simulink model "fymohukongzhifangzhen"  (R2012b)
settings: Solver=ode3  StartTime=0.0  StopTime=10.0  FixedStep=0.005  RelTol=1e-3
libraries: fuzblock x1
settings Model: Creator=Administrator  LastModifiedBy=Administrator

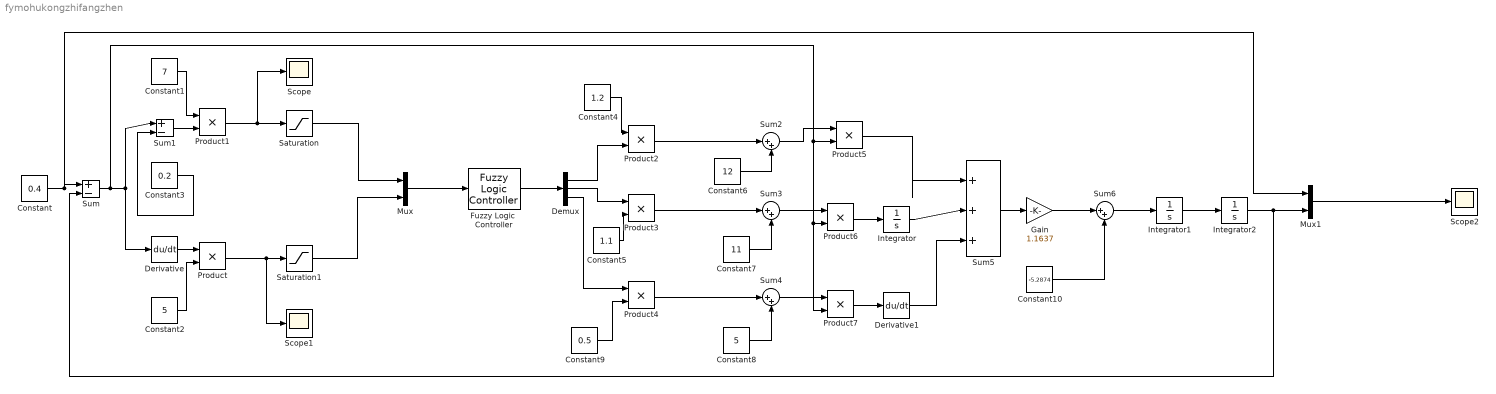
== system fymohukongzhifangzhen ==
  Constant : Constant  Value=0.4
  Constant1 : Constant  Value=7
  Constant10 : Constant  Value=-5.2874
  Constant2 : Constant  Value=5
  Constant3 : Constant  Value=0.2
  Constant4 : Constant  Value=1.2
  Constant5 : Constant  Value=1.1
  Constant6 : Constant  Value=12
  Constant7 : Constant  Value=11
  Constant8 : Constant  Value=5
  Constant9 : Constant  Value=0.5
  Demux : Demux  Outputs=3
  Derivative : Derivative
  Derivative1 : Derivative
  Fuzzy Logic  Controller : fuzblock/Fuzzy Logic  Controller  fis=Test
  Gain : Gain  Gain=1.1637
  Integrator : Integrator
  Integrator1 : Integrator
  Integrator2 : Integrator
  Mux : Mux  Inputs=2
  Mux1 : Mux  Inputs=2
  Product{,1..7} (8 alike) : Product  RndMeth=Zero
  Saturation : Saturate
  Saturation1 : Saturate
  Scope : Scope
  Scope1 : Scope
  Scope2 : Scope
      settings: SaveName=ScopeData2  MaxDataPoints=5000000
  Sum : Sum  Inputs=|+-
  Sum1 : Sum  Inputs=|+-
  Sum{2..4,6} (4 alike) : Sum  Inputs=|++
  Sum5 : Sum  Inputs=|+++
  wires:
  Derivative/1 -> Product/1
  Constant2/1 -> Product/2
  Constant/1 -> Mux1/1, Sum/1
  Sum/1 -> Product7/2, Product6/2, Product5/2, Sum1/1, Derivative/1
  Constant1/1 -> Product1/1
  Sum1/1 -> Product1/2
  Constant3/1 -> Sum1/2
  Product1/1 -> Scope/1, Saturation/1
  Product/1 -> Scope1/1, Saturation1/1
  Saturation/1 -> Mux/1
  Saturation1/1 -> Mux/2
  Mux/1 -> Fuzzy Logic  Controller/1
  Fuzzy Logic  Controller/1 -> Demux/1
  Demux/1 -> Product2/2
  Demux/2 -> Product3/1
  Demux/3 -> Product4/1
  Constant4/1 -> Product2/1
  Constant5/1 -> Product3/2
  Constant9/1 -> Product4/2
  Product2/1 -> Sum2/1
  Product3/1 -> Sum3/1
  Product4/1 -> Sum4/1
  Constant6/1 -> Sum2/2
  Constant7/1 -> Sum3/2
  Constant8/1 -> Sum4/2
  Sum2/1 -> Product5/1
  Sum3/1 -> Product6/1
  Sum4/1 -> Product7/1
  Product6/1 -> Integrator/1
  Product7/1 -> Derivative1/1
  Product5/1 -> Sum5/1
  Integrator/1 -> Sum5/2
  Derivative1/1 -> Sum5/3
  Sum5/1 -> Gain/1
  Gain/1 -> Sum6/1
  Constant10/1 -> Sum6/2
  Sum6/1 -> Integrator1/1
  Integrator1/1 -> Integrator2/1
  Integrator2/1 -> Sum/2, Mux1/2
  Mux1/1 -> Scope2/1
